simulink model "ufss_heading_cl"  (R2026a)
settings: Solver=ode45  StopTime=12  RelTol=1e-6
settings Model: Creator=musta  LastModifiedBy=musta

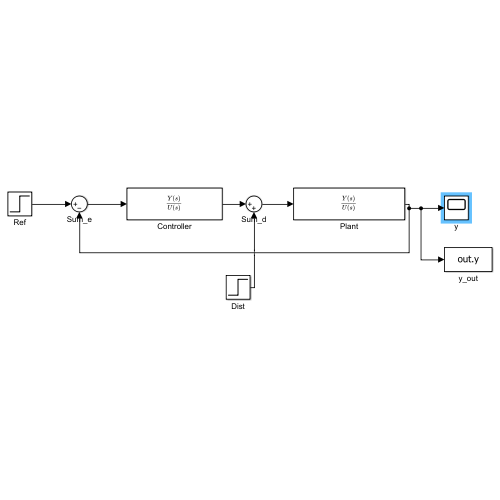
[thumbnail: Simulink's stored preview of the top-level diagram]
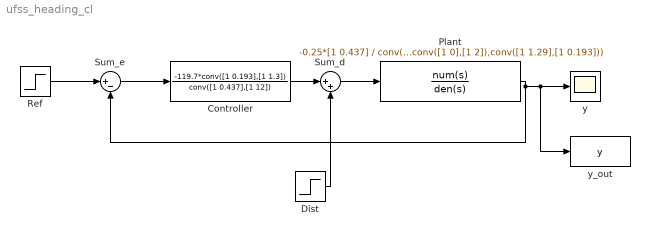
== system ufss_heading_cl ==
  Controller : TransferFcn  Numerator=-119.7*conv([1 0.193],[1 1.3])  Denominator=conv([1 0.437],[1 12])
  Dist : Step  Time=6  FinalValue=0  SampleTime=0
  Plant : TransferFcn  Numerator=-0.25*[1 0.437]  Denominator=conv(conv([1 0],[1 2]),conv([1 1.29],[1 0.193]))
  Ref : Step  Time=0  SampleTime=0
  Sum_d : Sum  Inputs=|++
  Sum_e : Sum  Inputs=|+-
  y : Scope
      settings: ActiveDisplayYMinimum=-1  ActiveDisplayYMaximum=1
  y_out : ToWorkspace  VariableName=y  SaveFormat=Timeseries  SampleTime=-1
  wires:
  Ref/1 -> Sum_e/1
  Sum_e/1 -> Controller/1
  Controller/1 -> Sum_d/1
  Dist/1 -> Sum_d/2
  Sum_d/1 -> Plant/1
  Plant/1 -> y/1, y_out/1, Sum_e/2
